simulink model "lin_controlsys_theta"  (R2019b)
settings: Solver=VariableStepAuto  StartTime=0.0  StopTime=5  RelTol=1e-3
values from neighbouring files (symbols this model uses):
  A = A*(v_phi(k,i)*s^i)    [Roberts_Q_design.m]    (also in main_fmincon.m = []; rocket_model.m = [0,1,0,0,0,0; ss_model.mat = [0  0; 1  0]; verif.m = [0,1;0,0])
  B = B*(s-alpha(i))    [Roberts_Q_design.m]    (also in controller_design.m = B*C(2); main_yp_fminunc.m = B*C(2); rocket_controllerdesign.m = B*C(2); rocket_controllerdesign_z.m = B*C(2))
  C = [0,1]    [controller_design.m]    (also in main_yp_fminunc.m; rocket_controllerdesign.m; rocket_controllerdesign_z.m; rocket_model.m = eye(6))
  K = minreal(Q/(1+Q*P))    [cost.m]    (also in cost_LQ.m = tf((conv(denQ{1},numK0{1})+conv(numQ{1},den_sys{1})),(conv(d; cost_con.m = tf((conv(denQ{1},numK0{1})+conv(numQ{1},den_sys{1})),(conv(d; cost_disturb.m = tf((conv(denQ{1},numK0{1})+conv(numQ{1},den_sys{1})),(conv(d; fminunc_LQ.m = tf((conv(denQ{1},numK0{1})+conv(numQ{1},den_sys{1})),(conv(d)
  Ts = 0.001    [main_rocketmodel.m]    (also in main_sim_rocket.m; sim_lin.m; square_sig.m; sum_squares_sig.m)
settings Model: Creator=bia  LastModifiedBy=bia
settings DataIOCC: ExternalInput=[ts, x_5]

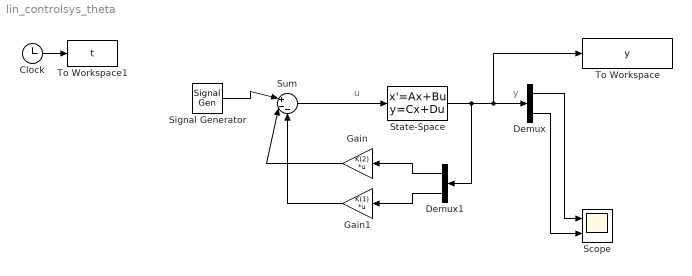
== system lin_controlsys_theta ==
  note: y
  note: u
  Clock : Clock
  Demux : Demux  Outputs=2
  Demux1 : Demux  Outputs=2
  Gain : Gain  Gain=K(2)  Multiplication=Matrix(K*u)
  Gain1 : Gain  Gain=K(1)  Multiplication=Matrix(K*u)
  Scope : Scope  NumInputPorts=2
  Signal Generator : SignalGenerator  WaveForm=square  Amplitude=1e-6  Units=rad/sec
  State-Space : StateSpace  A=A  B=B*C(2)  C=[0,1]  D=0  InitialCondition=[0; 0]
  Sum : Sum  Inputs=|+--
  To Workspace : ToWorkspace  VariableName=y  SampleTime=Ts
  To Workspace1 : ToWorkspace  VariableName=t  SampleTime=Ts
  wires:
  State-Space/1 -> Demux1/1, To Workspace/1, Demux/1
  Clock/1 -> To Workspace1/1
  Signal Generator/1 -> Sum/1
  Sum/1 -> State-Space/1
  Demux/1 -> Scope/1
  Demux/2 -> Scope/2
  Gain/1 -> Sum/2
  Demux1/2 -> Gain1/1
  Demux1/1 -> Gain/1
  Gain1/1 -> Sum/3
